simulink model "L16_AntiWindup"  (R2016b)
settings: Solver=ode1  StartTime=-5  StopTime=30  FixedStep=0.01  RelTol=1e-3
settings Model: Creator=Minkyun  LastModifiedBy=Minkyun

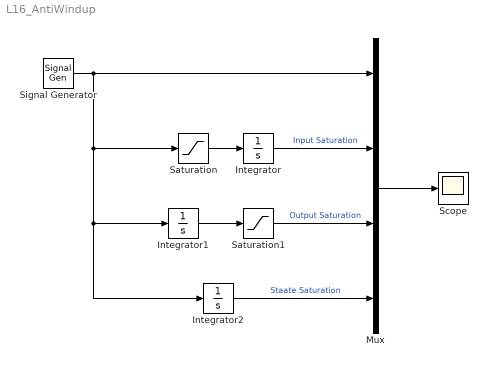
== system L16_AntiWindup ==
  Integrator : Integrator
  Integrator1 : Integrator
  Integrator2 : Integrator  LimitOutput=on  UpperSaturationLimit=0.5  LowerSaturationLimit=-0.5
  Mux : Mux
  Saturation : Saturate
  Saturation1 : Saturate
  Scope : Scope
  Signal Generator : SignalGenerator  WaveForm=square  Frequency=0.05
  wires:
  Mux/1 -> Scope/1
  Integrator2/1 -> Mux/4  "Staate Saturation"
  Integrator/1 -> Mux/2  "Input Saturation"
  Saturation/1 -> Integrator/1
  Signal Generator/1 -> Saturation/1, Integrator1/1, Integrator2/1, Mux/1
  Integrator1/1 -> Saturation1/1
  Saturation1/1 -> Mux/3  "Output Saturation"
